simulink model "IEEE_9bus"  (R2023b)
settings: Solver=ode23tb  StartTime=0.0  StopTime=1  FixedStep=Ts  RelTol=1e-3
values from neighbouring files (symbols this model uses):
  N = 1    [IEEE_9bus_calc.m]
  Ts = 50e-6    (= 5e-05)    [IEEE_9bus_calc.m]
  Ws = 2*pi*f    (= 376.991118431)    [IEEE_9bus_calc.m]
undefined symbols (not defined in the file or in its folder): D1, Delta, DiscIntNeverNeededParam, SM, SYS
libraries: spsLoadFlowBusLib x9, spsabctodq0Lib x7, spsThreePhasePISectionLineLib x6, spsExcitationSystemLib x6, spsGenericPowerSystemStabilizerLib x6, spsHydraulicTurbineandGovernorLib x6, spsMultiBandPowerSystemStabilizerLib x6, spsThreePhaseVIMeasurementLib x5, spsThreePhaseSeriesRLCLoadLib x4, DQN_Lib x3, spsGroundLib x3, spsThreePhaseParallelRLCBranchLib x3
(part 3 of 3)

== system IEEE_9bus/DQN_Mac1_V1/PQ ==
  note: PQ Measurement:
  note: Q = Vq*Id-Vd*Iq
  note: P = Vd*Id + Vq*Iq
  Iqd : Inport
  Vqd : Inport  Port=2
  Demux : Demux  Outputs=2
  Demux1 : Demux  Outputs=[1,1]
      settings: DisplayOption=none
  Gain : Gain  SaturateOnIntegerOverflow=on  OutDataTypeStr=Inherit: Same as input  ParamDataTypeStr=Inherit: Same as input
  Gain1 : Gain  SaturateOnIntegerOverflow=on  OutDataTypeStr=Inherit: Same as input  ParamDataTypeStr=Inherit: Same as input
  Product{2..5} (4 alike) : Product  InputSameDT=on  SaturateOnIntegerOverflow=on  OutDataTypeStr=Inherit: Same as first input
  Sum : Sum  InputSameDT=on  SaturateOnIntegerOverflow=on  OutDataTypeStr=Inherit: Same as first input
  Sum1 : Sum  Inputs=+-  InputSameDT=on  SaturateOnIntegerOverflow=on  OutDataTypeStr=Inherit: Same as first input
  Peo : Outport  VectorParamsAs1DForOutWhenUnconnected=off
  Qeo : Outport  Port=2  VectorParamsAs1DForOutWhenUnconnected=off
  wires:
  Demux1/2 -> Product4/2, Product3/2
  Demux/1 -> Product4/1, Product2/1
  Demux/2 -> Product5/1, Product3/1
  Sum1/1 -> Gain1/1  "Qeo"
  Sum/1 -> Gain/1  "Peo"
  Product5/1 -> Sum1/2
  Product4/1 -> Sum1/1
  Product3/1 -> Sum/2
  Product2/1 -> Sum/1
  Gain/1 -> Peo/1
  Gain1/1 -> Qeo/1
  Iqd/1 -> Demux1/1
  Demux1/1 -> Product2/2, Product5/2
  Vqd/1 -> Demux/1

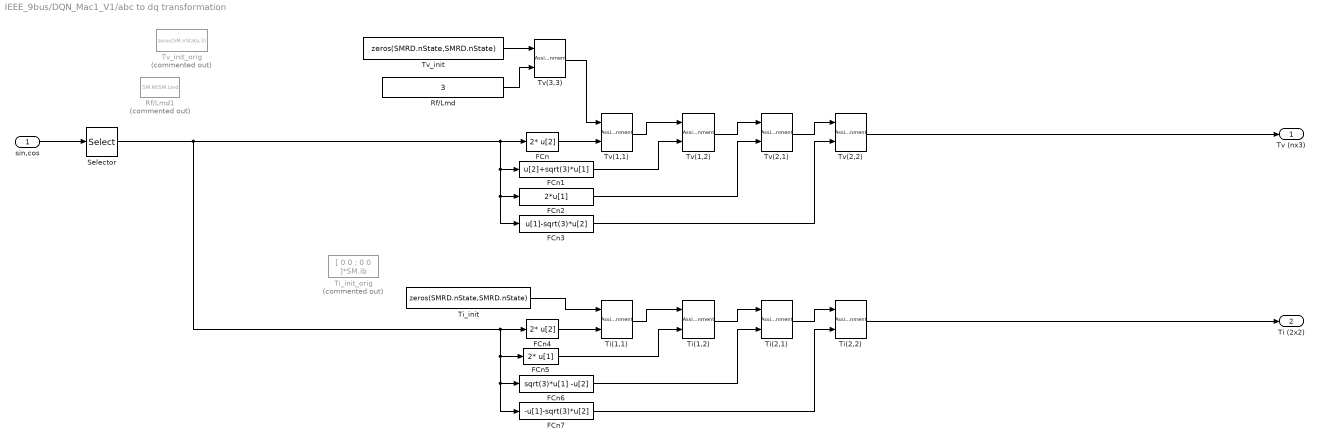
== system IEEE_9bus/DQN_Mac1_V1/abc to dq transformation ==
  sin,cos : Inport
  FCn : Fcn  Expr=2* u[2]  SampleTime=Ts
  FCn1 : Fcn  Expr=u[2]+sqrt(3)*u[1]  SampleTime=Ts
  FCn2 : Fcn  Expr=2*u[1]  SampleTime=Ts
  FCn3 : Fcn  Expr=u[1]-sqrt(3)*u[2]  SampleTime=Ts
  FCn4 : Fcn  Expr=2* u[2]  SampleTime=Ts
  FCn5 : Fcn  Expr=2* u[1]  SampleTime=Ts
  FCn6 : Fcn  Expr=sqrt(3)*u[1] -u[2]  SampleTime=Ts
  FCn7 : Fcn  Expr=-u[1]-sqrt(3)*u[2]  SampleTime=Ts
  Rf/Lmd : Constant  Value=3
  Rf/Lmd1 : Constant  Commented=on  Value=SM.Rf/SM.Lmd
  Selector : Selector  InputPortWidth=2  IndexOptions=Index vector (dialog)  Indices=[1 2]  OutputSizes=1
  "Ti(1,1) " : Assignment  NumberOfDimensions=2  DiagnosticForDimensions=Warning  IndexOptions=Index vector (dialog),Index vector (dialog)  Indices=1,1  OutputSizes=1,1
  "Ti(1,2) " : Assignment  NumberOfDimensions=2  DiagnosticForDimensions=Warning  IndexOptions=Index vector (dialog),Index vector (dialog)  Indices=1,2  OutputSizes=1,1
  "Ti(2,1) " : Assignment  NumberOfDimensions=2  DiagnosticForDimensions=Warning  IndexOptions=Index vector (dialog),Index vector (dialog)  Indices=2,1  OutputSizes=1,1
  "Ti(2,2) " : Assignment  NumberOfDimensions=2  DiagnosticForDimensions=Warning  IndexOptions=Index vector (dialog),Index vector (dialog)  Indices=2,2  OutputSizes=1,1
  Ti_init : Constant  Value=zeros(SMRD.nState,SMRD.nState)
  Ti_init_orig : Constant  Commented=on  Value="[ 0  0 ;  0  0  ]*SM.ib"
  Tv(1,1) : Assignment  NumberOfDimensions=2  DiagnosticForDimensions=Warning  IndexOptions=Index vector (dialog),Index vector (dialog)  Indices=1,1  OutputSizes=1,1
  Tv(1,2) : Assignment  NumberOfDimensions=2  DiagnosticForDimensions=Warning  IndexOptions=Index vector (dialog),Index vector (dialog)  Indices=1,2  OutputSizes=1,1
  Tv(2,1) : Assignment  NumberOfDimensions=2  DiagnosticForDimensions=Warning  IndexOptions=Index vector (dialog),Index vector (dialog)  Indices=2,1  OutputSizes=1,1
  Tv(2,2) : Assignment  NumberOfDimensions=2  DiagnosticForDimensions=Warning  IndexOptions=Index vector (dialog),Index vector (dialog)  Indices=2,2  OutputSizes=1,1
  Tv(3,3) : Assignment  NumberOfDimensions=2  DiagnosticForDimensions=Warning  IndexOptions=Index vector (dialog),Index vector (dialog)  Indices=3,3  OutputSizes=1,1
  Tv_init : Constant  Value=zeros(SMRD.nState,SMRD.nState)
  Tv_init_orig : Constant  Commented=on  Value=zeros(SM.nState,3)
  Tv (nx3) : Outport  VectorParamsAs1DForOutWhenUnconnected=off
  Ti (2x2) : Outport  Port=2  VectorParamsAs1DForOutWhenUnconnected=off
  wires:
  Tv(3,3)/1 -> Tv(1,1)/1
  Rf/Lmd/1 -> Tv(3,3)/2
  Tv_init/1 -> Tv(3,3)/1
  FCn7/1 -> "Ti(2,2) "/2
  "Ti(2,1) "/1 -> "Ti(2,2) "/1
  "Ti(1,2) "/1 -> "Ti(2,1) "/1
  FCn6/1 -> "Ti(2,1) "/2
  FCn5/1 -> "Ti(1,2) "/2
  "Ti(1,1) "/1 -> "Ti(1,2) "/1
  FCn4/1 -> "Ti(1,1) "/2
  FCn3/1 -> Tv(2,2)/2
  Tv(2,1)/1 -> Tv(2,2)/1
  Tv(1,2)/1 -> Tv(2,1)/1
  FCn2/1 -> Tv(2,1)/2
  FCn1/1 -> Tv(1,2)/2
  Tv(1,1)/1 -> Tv(1,2)/1
  FCn/1 -> Tv(1,1)/2
  sin,cos/1 -> Selector/1
  Ti_init/1 -> "Ti(1,1) "/1
  Selector/1 -> FCn7/1, FCn6/1, FCn5/1, FCn4/1, FCn/1, FCn1/1, FCn2/1, FCn3/1
  Tv(2,2)/1 -> Tv (nx3)/1
  "Ti(2,2) "/1 -> Ti (2x2)/1

== system IEEE_9bus/DQN_Mac1_V1/sin,cos ==
  theta : Inport
  Elementary Math : Trigonometry
  Elementary Math1 : Trigonometry  Operator=cos
  Mux3 : Mux  Inputs=2
  sin,cos : Outport  InitialOutput=0  VectorParamsAs1DForOutWhenUnconnected=off
  wires:
  theta/1 -> Elementary Math/1, Elementary Math1/1
  Elementary Math/1 -> Mux3/1
  Elementary Math1/1 -> Mux3/2
  Mux3/1 -> sin,cos/1

== system IEEE_9bus/DQN_Mac1_V1/Mechanical model1/Delay Prediction ==
  in : Inport
  F2 : Gain  Gain=2  SaturateOnIntegerOverflow=on  OutDataTypeStr=Inherit: Same as input  ParamDataTypeStr=Inherit: Same as input
  Sum1 : Sum  Inputs=+-  InputSameDT=on  SaturateOnIntegerOverflow=on  OutDataTypeStr=Inherit: Same as first input
  dw_delay : UnitDelay  InitialCondition=SMRD.dwo  SampleTime=SMRD.Ts  HasFrameUpgradeWarning=on
  dw_predict : UnitDelay  InitialCondition=SMRD.dwo  SampleTime=SMRD.Ts  HasFrameUpgradeWarning=on
  dw : Outport  VectorParamsAs1DForOutWhenUnconnected=off
  wires:
  dw_delay/1 -> dw_predict/1, F2/1
  in/1 -> dw_delay/1
  dw_predict/1 -> Sum1/2
  F2/1 -> Sum1/1
  Sum1/1 -> dw/1

== matlab function IEEE_9bus/MATLAB Function6 ==
  data: Vdq_vec input; Vs_c output; N parameter
function Vs_c   = fDQN012c(Vdq_vec, N)


    Vs_c  = complex(zeros(3, N+1));
    % Vr1_c = complex(zeros(3, N+1));
    % Vr2_c = complex(zeros(3, N+1));

    Vs_c(1,2)  = Vdq_vec(1) + 1i*Vdq_vec(2);
    % Vr1_c(1,2) = Vdq_vec(3) + 1i*Vdq_vec(4);
    % Vr2_c(1,2) = Vdq_vec(5) + 1i*Vdq_vec(6);



end

== matlab function IEEE_9bus/DQN_Mac1_V1/MATLAB Function2 ==
  data: Vdq_vec input; Vs_c output; N parameter
function Vs_c   = fDQN012c(Vdq_vec, N)


    Vs_c  = complex(zeros(3, N+1));
    % Vr1_c = complex(zeros(3, N+1));
    % Vr2_c = complex(zeros(3, N+1));

    Vs_c(1,2)  = Vdq_vec(1) + 1i*Vdq_vec(2);
    % Vr1_c(1,2) = Vdq_vec(3) + 1i*Vdq_vec(4);
    % Vr2_c(1,2) = Vdq_vec(5) + 1i*Vdq_vec(6);



end

== matlab function IEEE_9bus/Gain_DQNc_Mat4 ==
  data: Xpnz input; Ypnz output; Rabc parameter; chkInv parameter; HRM parameter
function Ypnz  = Gain_Mat2(Xpnz, Rabc, chkInv, HRM)
    persistent Rpnz;
    %persistent nrInp;
    persistent nrOut;

    mrows = size(Rabc,1)/3; %signal size
    mcols = size(Rabc,2)/3; %signal size

    nrInp = size(Rabc,1);

    % Ypnz = complex(zeros(nrInp, HRM+1));


    if(isempty(Rpnz)) 

        Rpnz = complex(zeros(3*mrows,3*mcols));
        a = -0.5+0.866i;
        a2 = -0.5-0.866i;
        Sas = [1,a,a2;1,a2,a;1,1,1]/3;
        %Ssa = eye(3)/(Sas);
        %nrInp = size(Xpnz,1) / 3;

        for i = 1 : mrows
            for j = 1 : mcols
                Rpnz((1:3) + (i-1)*3,(1:3) + (j-1)*3) = Sas*Rabc((1:3) + (i-1)*3,(1:3) + (j-1)*3)/Sas;
            end
        end

        if(chkInv)
            %Rpnz((1:3) + (i-1)*3,(1:3) + (j-1)*3) = eye(3)/Rpnz((1:3) + (i-1)*3,(1:3) + (j-1)*3);
            Rpnz = eye(3*mrows,3*mcols)/Rpnz;
        end

    end




    
    Ypnz = Rpnz*Xpnz;

end

== matlab function IEEE_9bus/DQn->ABC3 ==
  settings: updateMethod=DISCRETE
  data: Xdcpnz_c input; tho input; Xabc output; N parameter
%function abc = Mult(Z0,Zdp,Zqp,Zdn,Zqn,Zdz,Zqz,th, N)
function Xabc = dqn2abc(Xdcpnz_c,tho,N)

    persistent Sas;
    persistent Ssa;

    if(isempty(Sas)) 
        a = -0.5+0.866i;
        a2 = -0.5-0.866i;
        Sas = [1,a,a2;1,a2,a;1,1,1]/3;
        Ssa = eye(3)/(Sas);
    end

    Xabc = zeros(3,1);

    for i = 1 : N+1
    
    
        if(i>1)
            h = i-1;
    
            th = h*tho;
        
            mag_p = abs(Xdcpnz_c(1,i));
            ang_p = angle(Xdcpnz_c(1,i));
            mag_n = abs(Xdcpnz_c(2,i));
            ang_n = angle(Xdcpnz_c(2,i));
            mag_z = abs(Xdcpnz_c(3,i));
            ang_z = angle(Xdcpnz_c(3,i));
            
            abc3p = mag_p*[sin(th+ang_p) ; sin(th+ang_p-2*pi/3) ; sin(th+ang_p+2*pi/3) ];
            abc3n = mag_n*[sin(th+ang_n) ; sin(th+ang_n+2*pi/3) ; sin(th+ang_n-2*pi/3) ];
            abc3z = mag_z*[sin(th+ang_z) ; sin(th+ang_z)        ; sin(th+ang_z)  ];
        
            Xabc = Xabc + abc3p+abc3n+abc3z;
        else
            Xabc = Xabc + real(Ssa*(Xdcpnz_c(:,1)));
        
        end
    
        
    end

end

== matlab function IEEE_9bus/MATLAB Function5 ==
  data: Vdq_vec input; Vs_c output; N parameter
function Vs_c   = fDQN012c(Vdq_vec, N)


    Vs_c  = complex(zeros(3, N+1));
    % Vr1_c = complex(zeros(3, N+1));
    % Vr2_c = complex(zeros(3, N+1));

    Vs_c(1,2)  = Vdq_vec(1) + 1i*Vdq_vec(2);
    % Vr1_c(1,2) = Vdq_vec(3) + 1i*Vdq_vec(4);
    % Vr2_c(1,2) = Vdq_vec(5) + 1i*Vdq_vec(6);



end

== matlab function IEEE_9bus/Int_DQNc_Mat3 ==
  settings: updateMethod=DISCRETE
  data: Xpnz input; N parameter; dt parameter; w parameter; InitInt parameter; Zpnz output; R parameter; iL parameter; swFeed parameter
function Zpnz    = Int_DQN_Mat(Xpnz, N, dt, w, InitInt, R, iL, swFeed)


    nrSig = size(Xpnz,1)/3;
    Zpnz = complex(zeros(nrSig*3,N+1));

    persistent Zpnz_old;
    persistent Xpnz_old;
    persistent Krl1;
    persistent Krl2;
    persistent dt2;
        
    if(isempty(Zpnz_old)) 
    

        Zpnz_old = complex(zeros(nrSig*3,N+1));
        Xpnz_old = complex(zeros(nrSig*3,N+1));
        dt2 = dt/2;

        if(swFeed)
            mrows = size(R,1)/3; %signal size
            mcols = size(R,2)/3; %signal size

            szMatR = size(R,1);
            szMatiL = size(iL,1);

            if(szMatiL ~= szMatR || size(R,1) ~= size(R,2) || size(iL,1) ~= size(iL,2))
                error('[Int_DQN_Mat/swFeedback] check matrix sizes!');
            end
    
            Rpnz = complex(zeros(3*mrows,3*mcols));
            iLpnz = complex(zeros(3*mrows,3*mcols));

            a = -0.5+0.866i;
            a2 = -0.5-0.866i;
            Sas = [1,a,a2;1,a2,a;1,1,1]/3;
    
            for i = 1 : mrows
                for j = 1 : mcols
                     Rpnz((1:3) + (i-1)*3,(1:3) + (j-1)*3) = Sas*R((1:3) + (i-1)*3,(1:3) + (j-1)*3)/Sas;
                    iLpnz((1:3) + (i-1)*3,(1:3) + (j-1)*3) = Sas*iL((1:3) + (i-1)*3,(1:3) + (j-1)*3)/Sas;

                    Rpnz((1:3) + (i-1)*3,(1:3) + (j-1)*3) = diag(diag(real(Rpnz((1:3) + (i-1)*3,(1:3) + (j-1)*3))));
                    iLpnz((1:3) + (i-1)*3,(1:3) + (j-1)*3) = diag(diag(real(iLpnz((1:3) + (i-1)*3,(1:3) + (j-1)*3))));

                end
            end

            Rpnz = real(Rpnz);
            iLpnz = real(iLpnz);

            Krl1 = (iLpnz/(eye(szMatR)+dt2*Rpnz*iLpnz));
            Krl2 = (eye(szMatR)-dt2*Rpnz*iLpnz)/(eye(szMatR)+dt2*Rpnz*iLpnz);

        
            if(~isempty(InitInt))
                % Zpnz_old = x0;
                if(mod(numel(InitInt),3)~=0) error('[SS_DQNc_Mat] x0 vector with wrong size --> needs to be a multiple of 3!'); end
        
                for k = 1 : numel(InitInt)/3
                    Zpnz_old((k-1)*3+1:(k-1)*3+3,1) = Sas*InitInt((k-1)*3+1:(k-1)*3+3);
                end
            end



        else
            Krl1 = 1;
            Krl2 = 1;
        end
            
    end

    if(swFeed)
        Zpnz(:,1) = Krl1*dt2*(Xpnz(:,1)+Xpnz_old(:,1))+Krl2*Zpnz_old(:,1);
    else
        Zpnz(:,1) = dt2*(Xpnz(:,1)+Xpnz_old(:,1))+Zpnz_old(:,1);
    end

    Xpnz_old(:,1) = Xpnz(:,1);
    Zpnz_old(:,1) = Zpnz(:,1);

    for i = 1 : N
        if(N>0)
            wn =  i * w; 
            wndt2 = wn*dt2;

            A = 2*dt2/(1+wndt2^2);
            B = (1-wndt2^2)/(1+wndt2^2);

            if(swFeed)

                Zpnz(:,i+1) =      Krl1*A*(real(Xpnz(:,i+1))+wndt2*imag(Xpnz(:,i+1)))+Krl2*(B*real(Zpnz_old(:,i+1))+A*wn*imag(Zpnz_old(:,i+1))) ...
                             + 1i*(Krl1*A*(imag(Xpnz(:,i+1))-wndt2*real(Xpnz(:,i+1)))+Krl2*(B*imag(Zpnz_old(:,i+1))-A*wn*real(Zpnz_old(:,i+1))));
            else
                Zpnz(:,i+1) =      A*(real(Xpnz(:,i+1))+wndt2*imag(Xpnz(:,i+1)))+(B*real(Zpnz_old(:,i+1))+A*wn*imag(Zpnz_old(:,i+1))) ...
                             + 1i*(A*(imag(Xpnz(:,i+1))-wndt2*real(Xpnz(:,i+1)))+(B*imag(Zpnz_old(:,i+1))-A*wn*real(Zpnz_old(:,i+1))));
            end

            Zpnz_old(:,i+1) = Zpnz(:,i+1);

        end
    end


end

== matlab function IEEE_9bus/MATLAB Function1 ==
  data: Vdq_vec input; Vs_c output; N parameter
function Vs_c   = fDQN012c(Vdq_vec, N)


    Vs_c  = complex(zeros(3, N+1));
    % Vr1_c = complex(zeros(3, N+1));
    % Vr2_c = complex(zeros(3, N+1));

    Vs_c(1,2)  = Vdq_vec(1) + 1i*Vdq_vec(2);
    % Vr1_c(1,2) = Vdq_vec(3) + 1i*Vdq_vec(4);
    % Vr2_c(1,2) = Vdq_vec(5) + 1i*Vdq_vec(6);



end

== matlab function IEEE_9bus/MATLAB Function2 ==
  data: Vdq_vec input; Vs_c output; N parameter
function Vs_c   = fDQN012c(Vdq_vec, N)


    Vs_c  = complex(zeros(3, N+1));
    % Vr1_c = complex(zeros(3, N+1));
    % Vr2_c = complex(zeros(3, N+1));

    Vs_c(1,2)  = Vdq_vec(1) + 1i*Vdq_vec(2);
    % Vr1_c(1,2) = Vdq_vec(3) + 1i*Vdq_vec(4);
    % Vr2_c(1,2) = Vdq_vec(5) + 1i*Vdq_vec(6);



end

== matlab function IEEE_9bus/DQn->ABC1 ==
  settings: updateMethod=DISCRETE
  data: Xdcpnz_c input; tho input; Xabc output; N parameter
%function abc = Mult(Z0,Zdp,Zqp,Zdn,Zqn,Zdz,Zqz,th, N)
function Xabc = dqn2abc(Xdcpnz_c,tho,N)

    persistent Sas;
    persistent Ssa;

    if(isempty(Sas)) 
        a = -0.5+0.866i;
        a2 = -0.5-0.866i;
        Sas = [1,a,a2;1,a2,a;1,1,1]/3;
        Ssa = eye(3)/(Sas);
    end

    Xabc = zeros(3,1);

    for i = 1 : N+1
    
    
        if(i>1)
            h = i-1;
    
            th = h*tho;
        
            mag_p = abs(Xdcpnz_c(1,i));
            ang_p = angle(Xdcpnz_c(1,i));
            mag_n = abs(Xdcpnz_c(2,i));
            ang_n = angle(Xdcpnz_c(2,i));
            mag_z = abs(Xdcpnz_c(3,i));
            ang_z = angle(Xdcpnz_c(3,i));
            
            abc3p = mag_p*[sin(th+ang_p) ; sin(th+ang_p-2*pi/3) ; sin(th+ang_p+2*pi/3) ];
            abc3n = mag_n*[sin(th+ang_n) ; sin(th+ang_n+2*pi/3) ; sin(th+ang_n-2*pi/3) ];
            abc3z = mag_z*[sin(th+ang_z) ; sin(th+ang_z)        ; sin(th+ang_z)  ];
        
            Xabc = Xabc + abc3p+abc3n+abc3z;
        else
            Xabc = Xabc + real(Ssa*(Xdcpnz_c(:,1)));
        
        end
    
        
    end

end

== matlab function IEEE_9bus/MATLAB Function3 ==
  data: Vdq_vec input; Vs_c output; N parameter
function Vs_c   = fDQN012c(Vdq_vec, N)


    Vs_c  = complex(zeros(3, N+1));
    % Vr1_c = complex(zeros(3, N+1));
    % Vr2_c = complex(zeros(3, N+1));

    Vs_c(1,2)  = Vdq_vec(1) + 1i*Vdq_vec(2);
    % Vr1_c(1,2) = Vdq_vec(3) + 1i*Vdq_vec(4);
    % Vr2_c(1,2) = Vdq_vec(5) + 1i*Vdq_vec(6);



end

== matlab function IEEE_9bus/DQn->ABC2 ==
  settings: updateMethod=DISCRETE
  data: Xdcpnz_c input; tho input; Xabc output; N parameter
%function abc = Mult(Z0,Zdp,Zqp,Zdn,Zqn,Zdz,Zqz,th, N)
function Xabc = dqn2abc(Xdcpnz_c,tho,N)

    persistent Sas;
    persistent Ssa;

    if(isempty(Sas)) 
        a = -0.5+0.866i;
        a2 = -0.5-0.866i;
        Sas = [1,a,a2;1,a2,a;1,1,1]/3;
        Ssa = eye(3)/(Sas);
    end

    Xabc = zeros(3,1);

    for i = 1 : N+1
    
    
        if(i>1)
            h = i-1;
    
            th = h*tho;
        
            mag_p = abs(Xdcpnz_c(1,i));
            ang_p = angle(Xdcpnz_c(1,i));
            mag_n = abs(Xdcpnz_c(2,i));
            ang_n = angle(Xdcpnz_c(2,i));
            mag_z = abs(Xdcpnz_c(3,i));
            ang_z = angle(Xdcpnz_c(3,i));
            
            abc3p = mag_p*[sin(th+ang_p) ; sin(th+ang_p-2*pi/3) ; sin(th+ang_p+2*pi/3) ];
            abc3n = mag_n*[sin(th+ang_n) ; sin(th+ang_n+2*pi/3) ; sin(th+ang_n-2*pi/3) ];
            abc3z = mag_z*[sin(th+ang_z) ; sin(th+ang_z)        ; sin(th+ang_z)  ];
        
            Xabc = Xabc + abc3p+abc3n+abc3z;
        else
            Xabc = Xabc + real(Ssa*(Xdcpnz_c(:,1)));
        
        end
    
        
    end

end

== matlab function IEEE_9bus/MATLAB Function4 ==
  data: Vdq_vec input; Vs_c output; N parameter
function Vs_c   = fDQN012c(Vdq_vec, N)


    Vs_c  = complex(zeros(3, N+1));
    % Vr1_c = complex(zeros(3, N+1));
    % Vr2_c = complex(zeros(3, N+1));

    Vs_c(1,2)  = Vdq_vec(1) + 1i*Vdq_vec(2);
    % Vr1_c(1,2) = Vdq_vec(3) + 1i*Vdq_vec(4);
    % Vr2_c(1,2) = Vdq_vec(5) + 1i*Vdq_vec(6);



end

== matlab function IEEE_9bus/DQn->ABC4 ==
  settings: updateMethod=DISCRETE
  data: Xdcpnz_c input; tho input; Xabc output; N parameter
%function abc = Mult(Z0,Zdp,Zqp,Zdn,Zqn,Zdz,Zqz,th, N)
function Xabc = dqn2abc(Xdcpnz_c,tho,N)

    persistent Sas;
    persistent Ssa;

    if(isempty(Sas)) 
        a = -0.5+0.866i;
        a2 = -0.5-0.866i;
        Sas = [1,a,a2;1,a2,a;1,1,1]/3;
        Ssa = eye(3)/(Sas);
    end

    Xabc = zeros(3,1);

    for i = 1 : N+1
    
    
        if(i>1)
            h = i-1;
    
            th = h*tho;
        
            mag_p = abs(Xdcpnz_c(1,i));
            ang_p = angle(Xdcpnz_c(1,i));
            mag_n = abs(Xdcpnz_c(2,i));
            ang_n = angle(Xdcpnz_c(2,i));
            mag_z = abs(Xdcpnz_c(3,i));
            ang_z = angle(Xdcpnz_c(3,i));
            
            abc3p = mag_p*[sin(th+ang_p) ; sin(th+ang_p-2*pi/3) ; sin(th+ang_p+2*pi/3) ];
            abc3n = mag_n*[sin(th+ang_n) ; sin(th+ang_n+2*pi/3) ; sin(th+ang_n-2*pi/3) ];
            abc3z = mag_z*[sin(th+ang_z) ; sin(th+ang_z)        ; sin(th+ang_z)  ];
        
            Xabc = Xabc + abc3p+abc3n+abc3z;
        else
            Xabc = Xabc + real(Ssa*(Xdcpnz_c(:,1)));
        
        end
    
        
    end

end
